simulink model "RegenModelV1"  (R2015a)
settings: Solver=ode4  StartTime=0.0  StopTime=10  FixedStep=0.001  RelTol=1e-3
libraries: dsparch4 x1, simulink x1, dspsrcs4 x1
settings Model: CovModelRefEnable=off  Creator=Sven-VDR  LastModifiedBy=Alexander
settings DataIOCC: SaveFormat=Dataset
settings HardwareCC: ProdBitPerPointer=64  ProdLargestAtomicFloat=Float  ProdIntDivRoundTo=Zero  ProdEndianess=LittleEndian  ProdHWDeviceType=Specified
settings GRTTargetCC: GeneratePreprocessorConditionals=Use local settings

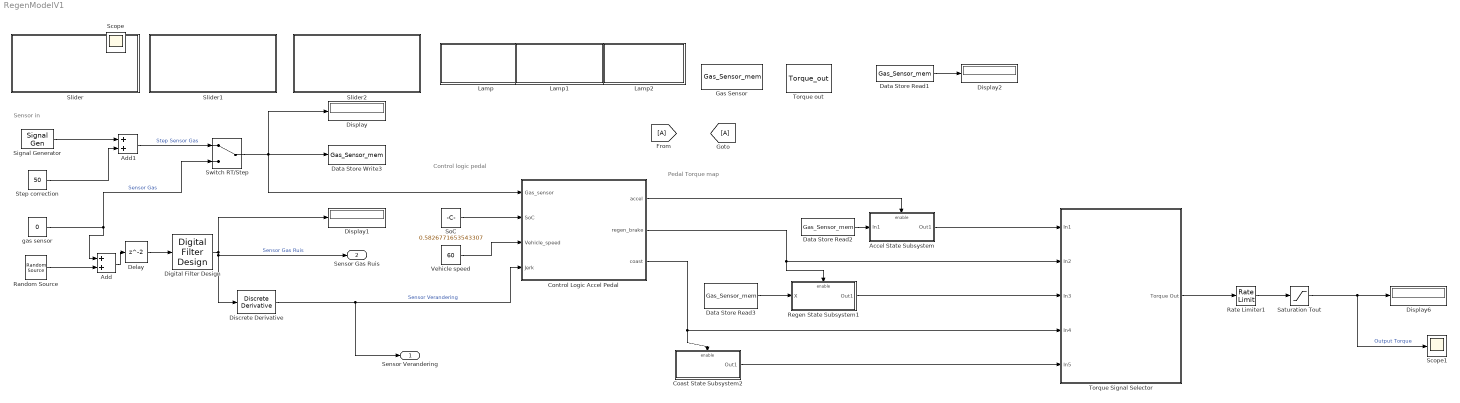
== system RegenModelV1 ==
  note: Pedal Torque map
  note: Control logic pedal
  note: Sensor in
  Accel State Subsystem : Subsystem  TreatAsAtomicUnit=on
  Add : Sum
  Add1 : Sum
  Coast State Subsystem2 : Subsystem  TreatAsAtomicUnit=on
  Control Logic Accel Pedal : Stateflow chart  TreatAsAtomicUnit=on
  Data Store Read1 : DataStoreRead  DataStoreName=Gas_Sensor_mem
  Data Store Read2 : DataStoreRead  DataStoreName=Gas_Sensor_mem
  Data Store Read3 : DataStoreRead  DataStoreName=Gas_Sensor_mem
  Data Store Write3 : DataStoreWrite  DataStoreName=Gas_Sensor_mem  SampleTime=0.001
  Delay : Delay  SampleTime=0.001
  Digital Filter Design : dsparch4/Digital Filter Design  mwdsp_browser_bugfix_var=off
  Discrete Derivative : simulink/Discrete/Discrete Derivative  gainval=1.0  ICPrevScaledInput=0.0  InputProcessing=Inherited  OutMin=[]  OutMax=[]  OutDataType=fixdt(1, 16)  OutScaling=2^-10  DoSatur=off
  Display{,1..2,6} (4 alike) : Display
  "Gas Sensor " : DataStoreMemory  DataStoreName=Gas_Sensor_mem  ReadBeforeWriteMsg=warning  WriteAfterWriteMsg=warning  WriteAfterReadMsg=warning
  Lamp : Subsystem  DialogController=hmiCreateDDGDialog  IsWebBlock=on  mask(MWDashboardBlock){webBlockId=e328b4f4-5e30-4047-a74c-6fdead431c46, webBlockType=lamp, ShowInLibBrowser=on, ShowInitialText=on, HMISrcModelName=RegenModelV1}
      mask prompts: webBlockType "WebBlock Type"; HMISrcModelName "Source Model"
      mask Help: helpview([docroot '/mapfiles/simulink.map'], 'hmi_lamp')
      mask Display:
      | if strcmp(get_param(bdroot(gcb),'BlockDiagramType'), 'library')
      |     image([(matlabroot) '/toolbox/simulink/hmi/icons/Lamp.png']);
      | end
  Lamp1 : Subsystem  DialogController=hmiCreateDDGDialog  IsWebBlock=on  mask(MWDashboardBlock){webBlockId=5aac5cf1-c578-4f64-997a-5f0bc1199dde, webBlockType=lamp, ShowInLibBrowser=on, ShowInitialText=on, HMISrcModelName=RegenModelV1}
      mask prompts: webBlockType "WebBlock Type"; HMISrcModelName "Source Model"
      mask Help: helpview([docroot '/mapfiles/simulink.map'], 'hmi_lamp')
      mask Display:
      | if strcmp(get_param(bdroot(gcb),'BlockDiagramType'), 'library')
      |     image([(matlabroot) '/toolbox/simulink/hmi/icons/Lamp.png']);
      | end
  Lamp2 : Subsystem  DialogController=hmiCreateDDGDialog  IsWebBlock=on  mask(MWDashboardBlock){webBlockId=30539f04-3b4b-48b4-ab88-6ba4f8a9e117, webBlockType=lamp, ShowInLibBrowser=on, ShowInitialText=on, HMISrcModelName=RegenModelV1}
      mask prompts: webBlockType "WebBlock Type"; HMISrcModelName "Source Model"
      mask Help: helpview([docroot '/mapfiles/simulink.map'], 'hmi_lamp')
      mask Display:
      | if strcmp(get_param(bdroot(gcb),'BlockDiagramType'), 'library')
      |     image([(matlabroot) '/toolbox/simulink/hmi/icons/Lamp.png']);
      | end
  Random Source : dspsrcs4/Random Source  SrcType=Uniform  NormMethod=Ziggurat  CltLength=12  MinVal=-1  MaxVal=1  MeanVal=0  VarVal=1  RepMode=Not repeatable  rawSeed=1  IsInherit=off  SampMode=Discrete  SampTime=0.001  SampFrame=1  DataType=Double  OutComplex=Real
  Rate Limiter1 : RateLimiter  RisingSlewLimit=100  FallingSlewLimit=-100  SampleTimeMode=inherited
  Regen State Subsystem1 : Subsystem  TreatAsAtomicUnit=on
  Saturation Tout : Saturate  UpperLimit=40  LowerLimit=-40
  Scope1 : Scope
      settings: YMin=-49.29204  YMax=43.62832
  Signal Generator : SignalGenerator  WaveForm=square  Amplitude=50  Frequency=0.25
  Slider : Subsystem  Description=Replaced Block  mask(Replaced Block){}
      mask help: This block has been replaced with an empty subsystem because it used functionality that is unavailable in Simulink R2015a.
      mask Display: fprintf('Replaced: %s\n','Dashboard Widget')
  Slider1 : Subsystem  Description=Replaced Block  mask(Replaced Block){}
      mask help: This block has been replaced with an empty subsystem because it used functionality that is unavailable in Simulink R2015a.
      mask Display: fprintf('Replaced: %s\n','Dashboard Widget')
  Slider2 : Subsystem  Description=Replaced Block  mask(Replaced Block){}
      mask help: This block has been replaced with an empty subsystem because it used functionality that is unavailable in Simulink R2015a.
      mask Display: fprintf('Replaced: %s\n','Dashboard Widget')
  SoC : Constant  Value=0.5826771653543307
  Step correction : Constant  Value=50
  Switch RT/Step : ManualSwitch
  Torque Signal Selector : Subsystem
  Torque out : DataStoreMemory  DataStoreName=Torque_out  ReadBeforeWriteMsg=warning  WriteAfterWriteMsg=warning  WriteAfterReadMsg=warning
  Vehicle speed : Constant  Value=60
  "gas sensor " : Constant  Value=0
  Sensor Verandering : Outport
  Sensor Gas Ruis : Outport  Port=2
  Scope : Scope
      settings: ShowLegends=on  YMin=-10  YMax=110
  wires:
  Discrete Derivative/1 -> Control Logic Accel Pedal/4(Jerk), Sensor Verandering/1  "Sensor Verandering"
  Delay/1 -> Digital Filter Design/1
  "gas sensor "/1 -> Switch RT/Step/2, Add/1  "Sensor Gas"
  Digital Filter Design/1 -> Display1/1, Sensor Gas Ruis/1, Discrete Derivative/1  "Sensor Gas Ruis"
  Add/1 -> Delay/1
  Control Logic Accel Pedal/2(regen_brake) -> Torque Signal Selector/2(In2), Regen State Subsystem1/Enable
  Control Logic Accel Pedal/3(coast) -> Torque Signal Selector/4(In4), Coast State Subsystem2/Enable
  Control Logic Accel Pedal/1(accel) -> Accel State Subsystem/Enable
  Data Store Read2/1 -> Accel State Subsystem/1(In1)
  Data Store Read1/1 -> Display2/1
  Data Store Read3/1 -> Regen State Subsystem1/1(X)
  Accel State Subsystem/1(Out1) -> Torque Signal Selector/1(In1)
  Regen State Subsystem1/1(Out1) -> Torque Signal Selector/3(In3)
  Coast State Subsystem2/1(Out1) -> Torque Signal Selector/5(In5)
  Torque Signal Selector/1(Torque Out) -> Rate Limiter1/1
  Rate Limiter1/1 -> Saturation Tout/1
  Saturation Tout/1 -> Display6/1, Scope1/1  "Output Torque"
  Switch RT/Step/1 -> Display/1, Data Store Write3/1, Control Logic Accel Pedal/1(Gas_sensor)
  Vehicle speed/1 -> Control Logic Accel Pedal/3(Vehicle_speed)
  SoC/1 -> Control Logic Accel Pedal/2(SoC)
  Random Source/1 -> Add/2
  Add1/1 -> Switch RT/Step/1  "Step Sensor Gas"
  Signal Generator/1 -> Add1/1
  Step correction/1 -> Add1/2

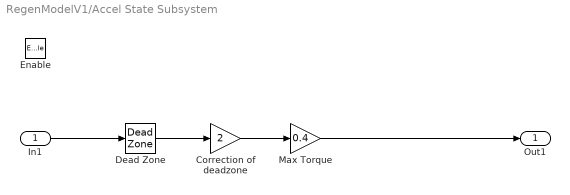
== system RegenModelV1/Accel State Subsystem ==
  In1 : Inport
  Enable : EnablePort
  "Correction of deadzone " : Gain  Gain=2
  Dead Zone : DeadZone  LowerValue=0  UpperValue=50  SaturateOnIntegerOverflow=on
  Max Torque : Gain  Gain=0.4
  Out1 : Outport
  wires:
  In1/1 -> Dead Zone/1
  Max Torque/1 -> Out1/1
  Dead Zone/1 -> "Correction of deadzone "/1
  "Correction of deadzone "/1 -> Max Torque/1

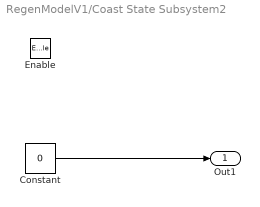
== system RegenModelV1/Coast State Subsystem2 ==
  Enable : EnablePort
  Constant : Constant  Value=0
  Out1 : Outport
  wires:
  Constant/1 -> Out1/1

== system RegenModelV1/Lamp ==

== system RegenModelV1/Lamp1 ==

== system RegenModelV1/Lamp2 ==

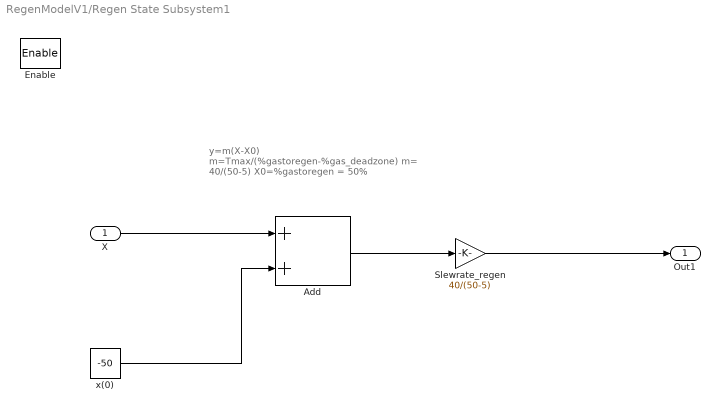
== system RegenModelV1/Regen State Subsystem1 ==
  note: y=m(X-X0)
      | m=Tmax/(%gastoregen-%gas_deadzone)
      | m= 40/(50-5)
      | X0=%gastoregen = 50%
  X : Inport
  Enable : EnablePort
  Add : Sum
  Slewrate_regen : Gain  Gain=40/(50-5)
  x(0) : Constant  Value=-50
  Out1 : Outport
  wires:
  X/1 -> Add/1
  x(0)/1 -> Add/2
  Add/1 -> Slewrate_regen/1
  Slewrate_regen/1 -> Out1/1

== system RegenModelV1/Slider ==

== system RegenModelV1/Slider1 ==

== system RegenModelV1/Slider2 ==

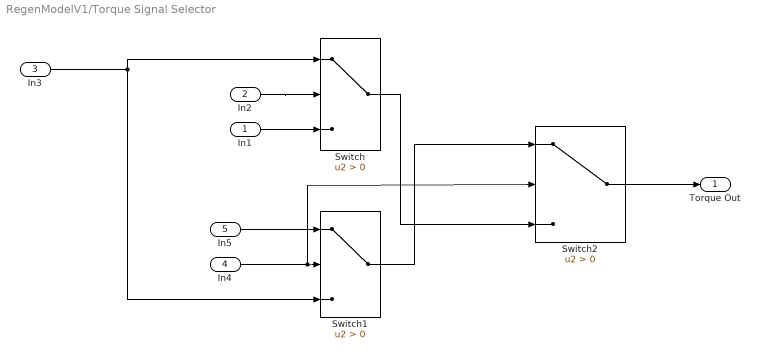
== system RegenModelV1/Torque Signal Selector ==
  In1 : Inport
  In2 : Inport  Port=2
  In3 : Inport  Port=3
  In4 : Inport  Port=4
  In5 : Inport  Port=5
  Switch : Switch  Criteria=u2 > Threshold
  Switch1 : Switch  Criteria=u2 > Threshold
  Switch2 : Switch  Criteria=u2 > Threshold
  Torque Out : Outport
  wires:
  In3/1 -> Switch1/3, Switch/1
  In1/1 -> Switch/3
  Switch1/1 -> Switch2/1
  In5/1 -> Switch1/1
  In4/1 -> Switch2/2, Switch1/2
  In2/1 -> Switch/2
  Switch2/1 -> Torque Out/1
  Switch/1 -> Switch2/3

== stateflow chart RegenModelV1/Control Logic Accel Pedal ==
  state Gas_pedal_logic
    state Coast
      entry: coast=1;
      entry: accel=0;
      entry: regen_brake=0;
      entry: BrakeFlag=0;
    state Accel
      entry: accel=1;
      entry:regen_brake=0;
      entry: coast =0;
    state RegenBrake
      entry: regen_brake=1;
      entry: accel=0;
      entry: coast=0;
      entry: BrakeFlag=0;
    Accel -> Coast [order 2] : [BrakeFlag==1 && (Vehicle_speed<10 || SoC>0.95)]
    Coast -> Accel [order 1] : [BrakeFlag==0 && Gas_sensor>50 && Jerk>3]
    (default) -> Accel : {BrakeFlag=0;}
    Coast -> RegenBrake [order 2] : [Vehicle_speed>10 && SoC<0.95]
    RegenBrake -> Coast [order 2] : [SoC>0.95]
    RegenBrake -> Coast [order 1] : [Vehicle_speed<10]
    Accel -> (junction 277) [order 3] : [Gas_sensor>50]
    (junction 277) -> Accel : {BrakeFlag=1;}
    RegenBrake -> Accel [order 3] : [BrakeFlag==0&& Gas_sensor>50]
    Accel -> RegenBrake [order 1] : [BrakeFlag==1 &&Gas_sensor<50]
  data: Gas_sensor input; SoC input; accel output; regen_brake output; coast output; Vehicle_speed input; BrakeFlag local; Jerk input
